simulink model "satelita"  (R2024a)
settings: Solver=ode4  StartTime=0.0  StopTime=10.0  FixedStep=2^-7  RelTol=1e-3
libraries: simulink x1
settings Model: Creator=zv53855  LastModifiedBy=zv53855

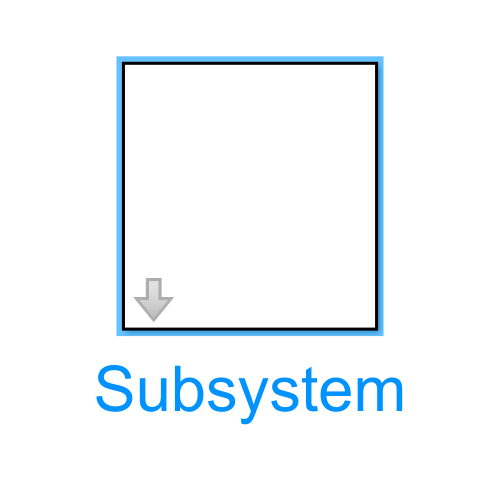
[thumbnail: Simulink's stored preview of the top-level diagram]
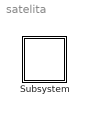
== system satelita ==
  Subsystem : Subsystem  mask{G=9.81, R=3, Rs=0.2, M=250, x0=3, y0=7, Vx0=17, Vy0=0}
      mask prompts: G "gravitation"; R "planet radius"; Rs "satellite radius"; M "planet mass"; x0 "x"; y0 "y"; Vx0 "velocity x"; Vy0 "velocity y"

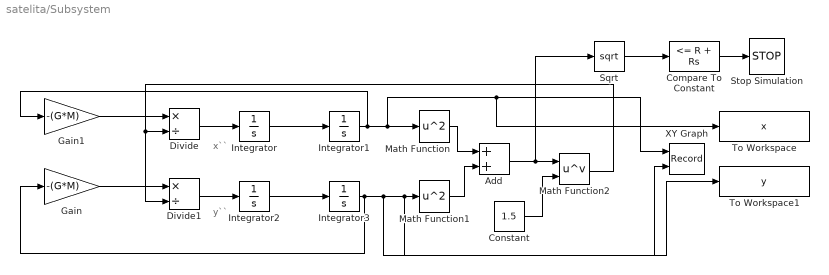
== system satelita/Subsystem ==
  note: y``
  note: x``
  Add : Sum
  Compare To Constant : simulink/Logic and Bit Operations/Compare To Constant  relop=<=  const=R + Rs  OutDataTypeStr=boolean
  Constant : Constant  Value=1.5
  Divide : Product  Inputs=*/
  Divide1 : Product  Inputs=*/
  Gain : Gain  Gain=-(G*M)
  Gain1 : Gain  Gain=-(G*M)
  Integrator : Integrator  InitialCondition=Vx0
  Integrator1 : Integrator  InitialCondition=x0
  Integrator2 : Integrator  InitialCondition=Vy0
  Integrator3 : Integrator  InitialCondition=y0
  Math Function : Math  Operator=square
  Math Function1 : Math  Operator=square
  Math Function2 : Math  Operator=pow
  Sqrt : Sqrt
  Stop Simulation : Stop
  To Workspace : ToWorkspace  VariableName=x  SampleTime=-1
  To Workspace1 : ToWorkspace  VariableName=y  SampleTime=-1
  XY Graph : Record  FileSettingsInternal="{\"entries\":[{\"content\":{\"excelSettings\":{\"content\":{},\"type\":\"Streamout.ExcelSettings\"}},\"type\":\"Streamout.FileSettingStorage\",\"uuid\":\"\"}],\"packageUris\":[\"http:\\/\\/schema.mathworks.com\\/mf0\\/streamout_blocks\\/R2020a\"],\"version\":\"1.0\"}"  Layout=[1 1]  SignalsInternal="{\"entries\":[{\"content\":{\"signals\":[{\"content\":{\"blockPath\":[],\"dimensions\":[1],\"domain\":\"\",\"lineColor\":\"#a2142f\",\"plots\":[ 1 ],\"port\":1,\"sid\":[\"\"],\"signalID\":1,\"signalName\":\"Integrator1\"},\"type\":\"RecordBlkView.Signal\",\"uuid\":\"\"},{\"content\":{\"blockPath\":[],\"dimensions\":[1],\"domain\":\"\",\"lineColor\":\"#139fff\",\"plots\":[ 1 ],\"port\":2,\"sid\":[\"\"],\"signalID\":2,\"signalName\":\"Integrator3\"},\"type\":\"RecordBlkView.Signal\",\"uuid\":\"\"}]},\"type\":\"RecordBlkView.InputSignals\",\"uuid\":\"\"}],\"packageUris\":[\"http:\\/\\/schema.mathworks.com\\/mf0\\/streamout_blocks\\/R2020a\"],\"version\":\"1.0\"}"  VisualizationBindings="{\"xyplotplugin\":{\"info\":[{\"series\":[{\"bindingParametersList\":[{\"parameter\":\"X-Axis\",\"signalID\":1,\"signalName\":\"Integrator1\"},{\"parameter\":\"Y-Axis\",\"signalID\":2,\"signalName\":\"Integrator3\"}],\"seriesID\":0}],\"subplotID\":1}]}}"  CompatibilityTag=XY
  wires:
  Math Function2/1 -> Divide1/2, Divide/2
  Integrator2/1 -> Integrator3/1
  Integrator/1 -> Integrator1/1
  Divide1/1 -> Integrator2/1
  Gain/1 -> Divide1/1
  Divide/1 -> Integrator/1
  Integrator3/1 -> Gain/1, XY Graph/2, To Workspace1/1, Math Function1/1
  Integrator1/1 -> Gain1/1, XY Graph/1, To Workspace/1, Math Function/1
  Math Function1/1 -> Add/2
  Math Function/1 -> Add/1
  Constant/1 -> Math Function2/2
  Add/1 -> Sqrt/1, Math Function2/1
  Gain1/1 -> Divide/1
  Compare To Constant/1 -> Stop Simulation/1
  Sqrt/1 -> Compare To Constant/1
